simulink model "Masse_MultirotorSimHinf"  (R2018b)
settings: Solver=VariableStepAuto  StartTime=0.0  StopTime=Simulation.T_END  MaxStep=Simulation.TS_MAX  RelTol=1e-3  EnableMultiTasking=on
PreLoadFcn:
  | % InitializeParameters;
undefined symbols (not defined in the file): Aero, armed, ctrl_state, INIT_PARAM_VECTOR, Initial, K_i, K_p, Motor, mpc_att_sp, mpc_ctrl_state, mpc_manual, mpc_pos_sp_triplet, mpc_vehicle_land_detected, mpc_vehicle_status, Simulation, SOF1, SOF2, Uav, Upsilon, v_att_sp, v_control_mode
libraries: simulink_extras x9, simulink x6, dspstat3 x1, Px4Library x1
(part 1 of 11)
settings Model: PauseTimes=10.09  Creator=jban039  LastModifiedBy=jban039
settings DataIOCC: Decimation=10  ReturnWorkspaceOutputs=on  OutputOption=SpecifiedOutputTimes  OutputTimes=Simulation.T_OUT
settings OptimizationCC: LifeSpan=inf
settings DebuggingCC: ReadBeforeWriteMsg=DisableAll  WriteAfterWriteMsg=DisableAll  WriteAfterReadMsg=DisableAll  MultiTaskDSMMsg=none  UnconnectedLineMsg=none  AllowSymbolicDim=off  SFUnexpectedBacktrackingDiag=warning  SFNoUnconditionalDefaultTransitionDiag=warning  SFExecutionAtInitializationDiag=none
settings ModelReferenceCC: UpdateModelReferenceTargets=IfOutOfDate  ModelReferenceMinAlgLoopOccurrences=on  PropagateSignalLabelsOutOfModel=off
settings SFSimCC: SFSimEcho=off  SimUseLocalCustomCode=off
settings RTWCC: RTWUseLocalCustomCode=off
settings CodeAppCC: StateflowObjectComments=on
settings GRTTargetCC: TargetLangStandard=C89/C90 (ANSI)
settings ConfigComp: CovMetricSettings=dw  CovHtmlReporting=on  CovSaveCumulativeToWorkspaceVar=on  CovSaveSingleToWorkspaceVar=on  CovExternalEMLEnable=off

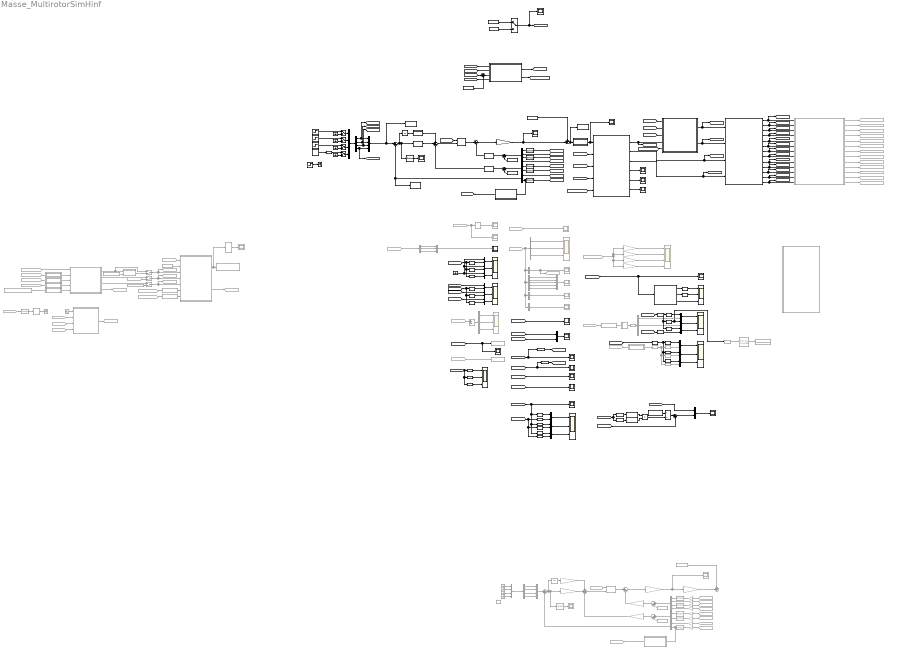
== system Masse_MultirotorSimHinf ==
  note: Important Notes
      |
      | NWU coordinate system used, therefore xBody faces forward, yBody faces to the left and zBody faces up
      | The UAV's state estimator, an extended kalman filter (referred to as LPE), is used for 3D position and velocity states.
      | PX4 rotor assignment: 1: front right, 2: back left, 3: front left, 4: back right
  note: Variables Description
      |
      | Variable
      | Vector notation
      | Frame
      | Description
      |
      | xi
      | [x y z]
      | World
      | Position
      |
      | eta
      | [phi theta psi]
      | World
      | Roll pitch yaw orientation
      |
      | nuBody
      | [p q r]
      | Body
      | Angular velocity
      |
      | q
      | [q1 q2 q3 q4]
      | World
      | Quaternion orientation
      |
      | Uav.BETA
      | [beta1 ... betaN]
      | Body
      | Angle to motor (CCW)
  note: Applied wind speed
  note: Inputs
  note: Scopes
  Acc : Scope  NumInputPorts=3
  Actuator controls : Scope  Commented=on
  Add : Sum  Commented=on  Inputs=+-
  Angular moments : Scope  NumInputPorts=3
  Angular rate integral : Scope  Commented=on  NumInputPorts=3
  Angular rates : Scope  NumInputPorts=3
  Applied body velocity : Scope
  Applied motor velocity : Scope  Commented=on  NumInputPorts=4
  Applied wind speed : Subsystem
  Attitude : Scope  NumInputPorts=3
  Attitude (quat) : Scope  Commented=on
  Bus Selector1 : BusSelector  Commented=on  OutputSignals=rates_sp
  Bus Selector10 : BusSelector  Commented=on  OutputSignals=mpc_local_pos_sp.acc_x,mpc_local_pos_sp.acc_y,mpc_local_pos_sp.acc_z
  Bus Selector2 : BusSelector  Commented=on  OutputSignals=controller_status.roll_rate_integ,controller_status.pitch_rate_integ,controller_status.yaw_rate_integ
  Bus Selector3 : BusSelector  Commented=on  OutputSignals=v_control_mode.flag_control_attitude_enabled,v_control_mode.flag_control_auto_enabled,v_control_mode.flag_control_manual_enabled,v_control_mode.flag_control_rates_enabled,v_control_mode.flag_control_velocity_enabled
  Bus Selector4 : BusSelector  Commented=on  OutputSignals=ctrl_state.q
  Bus Selector6 : BusSelector  Commented=on  OutputSignals=actuators.control
  Compute Sph : MATLAB Function  TreatAsAtomicUnit=on
  Constant : Constant  Value=Initial.U_M
  Constant1 : Constant  Value=abs(Uav.G(3))
  Constant2 : Constant  Value=Initial.Y2
  Constant3 : Constant  Value=Initial.Y1
  Constant4 : Constant  Commented=on  Value=Initial.U_M
  Constant5 : Constant  Commented=on  Value=Initial.Y2
  Constant6 : Constant  Commented=on  Value=Initial.Y1
  Default control stick positions : Constant  Commented=on  Value=[0; 0; 0.5; 0]
  Degrees to Radians : simulink_extras/Transformations/Degrees to Radians
  Degrees to Radians1 : simulink_extras/Transformations/Degrees to Radians  Commented=on
  Delay1 : Delay  Commented=on  DelayLength=1  SampleTime=1/10
  Demux : Demux  Commented=on  Outputs=3
  Demux1 : Demux
  Demux3 : Demux  Commented=on
  Demux6 : Demux  Commented=on  Outputs=3
  Desired accelerations : Scope
  Desired euler angles : Scope  Commented=on
  Desired quaternion : Scope  Commented=on
  Desired thrust : Scope  Commented=on
  Desired yaw rate : Scope
  Display : Display  Commented=on
  Divide : Product  Inputs=*/
  Divide1 : Product  Inputs=**
  Drag forces : Scope
  Drag model : ModelReference  ModelNameDialog=DragModelAIAAv3  SimulationMode=Normal  ModelReferenceVersion=1.368
  Drag moments : Scope
  Drag moments1 : Scope
  Fcn : Fcn  Expr=cos(u)
  Fcn1 : Fcn  Expr=cos(u)
  Fixed wind input : Constant  Value=[5.000000; 0.000000; 0]
  Flags : Scope  Commented=on
  From14 : From  Commented=on  GotoTag=attRateSp
  From16 : From  Commented=on  GotoTag=thrustDes
  From20 : From  Commented=on  GotoTag=posCtrlBus
  From21 : From  Commented=on  GotoTag=attCtrlBus
  From22 : From  Commented=on  GotoTag=qDes
  From34 : From  Commented=on  GotoTag=qDes
  From37 : From  Commented=on  GotoTag=VMotor_appBody
  From49 : From  Commented=on  GotoTag=R_star_bi
  From50 : From  Commented=on  GotoTag=xi
  From51 : From  Commented=on  GotoTag=eta
  From52 : From  Commented=on  GotoTag=xi
  From53 : From  Commented=on  GotoTag=xiDot
  From54 : From  Commented=on  GotoTag=nuBody
  From55 : From  Commented=on  GotoTag=xi
  From56 : From  Commented=on  GotoTag=xiDot
  From57 : From  Commented=on  GotoTag=eta
  From7 : From  Commented=on  GotoTag=eta
  From8 : From  Commented=on  GotoTag=xiMeasured
  Gain : Gain  Commented=on  Gain=[1;0;0;0]  Multiplication=Matrix(u*K)
  Gain1 : Gain  Commented=on  Gain=[0;1;0;0]  Multiplication=Matrix(u*K)
  Gain2 : Gain  Commented=on  Gain=[0;0;1;0]  Multiplication=Matrix(u*K)
  Gain3 : Gain  Commented=on  Gain=[0;0;0;1]  Multiplication=Matrix(u*K)
  Goto13 : Goto  Commented=on  GotoTag=VBodyMeasured
  Goto14 : Goto  Commented=on  GotoTag=VBodyDotMeasured
  Goto15 : Goto  Commented=on  GotoTag=qMeasured
  Goto16 : Goto  Commented=on  GotoTag=qDotMeasured
  Goto17 : Goto  Commented=on  GotoTag=qDDotMeasured
  Goto18 : Goto  Commented=on  GotoTag=nuBodyMeasured
  Goto19 : Goto  Commented=on  GotoTag=nuBodyDotMeasured
  Goto20 : Goto  Commented=on  GotoTag=xiMeasured
  Goto21 : Goto  Commented=on  GotoTag=xiDotMeasured
  Goto22 : Goto  Commented=on  GotoTag=xiDDotMeasured
  Goto23 : Goto  Commented=on  GotoTag=etaMeasured
  Goto24 : Goto  Commented=on  GotoTag=etaDotMeasured
  Goto25 : Goto  Commented=on  GotoTag=etaDDotMeasured
  Goto27 : Goto  Commented=on  GotoTag=R_star_bi
  Goto28 : Goto  Commented=on  GotoTag=attRateSp
  Ground{,5..8} (5 alike) : Ground  Commented=on
  Ground{1..4,9} (5 alike) : Ground
  Integrator1 : Integrator  Commented=on
  Integrator6 : Integrator
  K_i : Subsystem
      mask Display: fprintf('K_i')
  K_p : Subsystem
      mask Display: fprintf('K_p')
  Ki1 : Gain  Commented=on  Gain=K_i  Multiplication=Matrix(K*u)
  Kp1 : Gain  Commented=on  Gain=K_p  Multiplication=Matrix(K*u)
  Logging buffer : Subsystem
  MATLAB Function : MATLAB Function  TreatAsAtomicUnit=on
  MATLAB Function1 : MATLAB Function  Commented=on  TreatAsAtomicUnit=on
  Manual Switch{,1..3} (4 alike) : ManualSwitch
  Motor model : ModelReference  ModelNameDialog=MotorModelAIAAv3  SimulationMode=Normal  ModelReferenceVersion=1.394
  Motors - NED to NWU1 : Gain  Commented=on  Gain=[0 0 0 1; 0 0 1 0; 0 1 0 0; 1 0 0 0]  Multiplication=Matrix(K*u)
  Moving Average : dspstat3/Moving Average  Commented=on  Method=Sliding window  ForgettingFactorPort=off  SpecifyWindowLength=on  WindowLength=500  ForgettingFactor=0.9  SimulateUsing=Code generation
  Mux{,1,3,5..18,20..21} (19 alike) : Mux  Inputs=2
  Mux19 : Mux
  Mux2 : Mux  Commented=on  Inputs=5
  Mux22 : Mux
  Mux23 : Mux
  Mux24 : Mux  Commented=on  Inputs=2
  Mux25 : Mux  Commented=on
  Mux26 : Mux  Commented=on  Inputs=2
  Mux27 : Mux  Commented=on
  Mux28 : Mux  Commented=on
  Mux4 : Mux  Commented=on  Inputs=3
  NWU to NED Position1 : Subsystem  Commented=on  AncestorBlock=Px4Library/NWU to NED Position  mask(Coordinate transform){}
      mask help:
      | Convert a 3x1 vector or 4x1 quaternion from a North West Up to a North East Down coordinate system.
      |
      | The appropriate coordinate transform is automatically selected based on the input size.
  NWU to NED Quaternion3 : Subsystem  Commented=on  AncestorBlock=Px4Library/NWU to NED Quaternion  mask(Coordinate transform){}
      mask help:
      | Convert a 3x1 vector or 4x1 quaternion from a North West Up to a North East Down coordinate system.
      |
      | The appropriate coordinate transform is automatically selected based on the input size.
  NWU to NED{8..15} (8 alike) : Gain  Commented=on  Gain=[1 0 0; 0 -1 0; 0 0 -1]  Multiplication=Matrix(K*u)
  Omega : Scope
  Position tracking : Scope  NumInputPorts=3
  Product : Product  Multiplication=Matrix(*)
  Product1 : Product  Commented=on  Multiplication=Matrix(*)
  Quadcopter mixer : Px4Library/Quadcopter mixer  Commented=on  MC_SAMPLING_PERIOD=0.002
  Quadrotor Euler Model : Subsystem  Commented=on
  Quadrotor Quaternion Model : Subsystem
  Quaternion to Euler Angles : Subsystem  Commented=on  AncestorBlock=QuaternionLibrary/Quaternion to Euler Angles
      mask help: Convert an orientation quaternion to a vector of Euler angles
      mask Help:
      | Convert an orientation quaternion
      | [q1 q2 q3 q4]
      | where:
      | - q1 is the rotation in radians
      | - [q2 q3 q4] is the vector around which the rotation is performed)
      | to a vector of Euler angles
      | [roll, pitch, yaw]
      | Based on code from the PX4 firmware: https://github.com/PX4/Firmware
      mask Display: disp('Q2E')
  Quaternion to Euler Angles1 : Subsystem  Commented=on  AncestorBlock=QuaternionLibrary/Quaternion to Euler Angles
      mask help: Convert an orientation quaternion to a vector of Euler angles
      mask Help:
      | Convert an orientation quaternion
      | [q1 q2 q3 q4]
      | where:
      | - q1 is the rotation in radians
      | - [q2 q3 q4] is the vector around which the rotation is performed)
      | to a vector of Euler angles
      | [roll, pitch, yaw]
      | Based on code from the PX4 firmware: https://github.com/PX4/Firmware
      mask Display: disp('Q2E')
  Radians to Degrees{1..2,4..5,7} (5 alike) : simulink_extras/Transformations/Radians to Degrees
  Radians to Degrees3 : simulink_extras/Transformations/Radians to Degrees  Commented=on
  Radians to Degrees6 : simulink_extras/Transformations/Radians to Degrees  Commented=on
  Ramp : simulink/Sources/Ramp  slope=5  start=0  InitialOutput=0
  Rate setpoints : Scope  Commented=on
  SOF1 : Subsystem
      mask Display: fprintf('SOF1')
  SOF2 : Subsystem
      mask Display: fprintf('SOF2')
  SOF3 : Gain  Commented=on  Gain=SOF1  Multiplication=Matrix(K*u)
  SOF4 : Gain  Commented=on  Gain=SOF2  Multiplication=Matrix(K*u)
  Scope : Scope
  Scope1 : Scope  Commented=on
  Select Thrust : Selector  InputPortWidth=3  IndexOptions=Index vector (dialog)  Indices=[3]  OutputSizes=1
  Select pitch : Selector  InputPortWidth=3  IndexOptions=Index vector (dialog)  Indices=2  OutputSizes=1
  Select roll : Selector  InputPortWidth=3  IndexOptions=Index vector (dialog)  Indices=1  OutputSizes=1
  Select z : Selector  InputPortWidth=3  IndexOptions=Index vector (dialog)  Indices=[3]  OutputSizes=1
  Selector{,3,6,9,15,23..24} (7 alike) : Selector  InputPortWidth=3  IndexOptions=Index vector (dialog)  Indices=1  OutputSizes=1
  Selector{1,4,7,10,16,19,21} (7 alike) : Selector  InputPortWidth=3  IndexOptions=Index vector (dialog)  Indices=2  OutputSizes=1
  Selector{2,5,8,11,17,20,22,25,28..29} (10 alike) : Selector  InputPortWidth=3  IndexOptions=Index vector (dialog)  Indices=3  OutputSizes=1
  Selector12 : Selector  Commented=on  InputPortWidth=3  IndexOptions=Index vector (dialog)  Indices=2  OutputSizes=1
  Selector{13,31,34..35} (4 alike) : Selector  Commented=on  InputPortWidth=3  IndexOptions=Index vector (dialog)  Indices=3  OutputSizes=1
  Selector14 : Selector  Commented=on  InputPortWidth=3  IndexOptions=Index vector (dialog)  Indices=1  OutputSizes=1
  Selector18 : Selector  Commented=on  InputPortWidth=8  IndexOptions=Index vector (dialog)  Indices=[1 2 3]  OutputSizes=1
  Selector26 : Selector  InputPortWidth=3  IndexOptions=Index vector (dialog)  Indices=[2 1]  OutputSizes=1
  Selector27 : Selector  InputPortWidth=3  IndexOptions=Index vector (dialog)  Indices=[2 1]  OutputSizes=1
  Selector30 : Selector  InputPortWidth=4  IndexOptions=Index vector (dialog)  Indices=4  OutputSizes=1
  Selector32 : Selector  Commented=on  InputPortWidth=3  IndexOptions=Index vector (dialog)  Indices=[2 1]  OutputSizes=1
  Selector33 : Selector  Commented=on  InputPortWidth=3  IndexOptions=Index vector (dialog)  Indices=[2 1]  OutputSizes=1
  Selector36 : Selector  Commented=on  InputPortWidth=4  IndexOptions=Index vector (dialog)  Indices=4  OutputSizes=1
  Sensor Model : Subsystem  Commented=on
  Spherical body velocity : Scope  NumInputPorts=3
  Step : Step  Time=10  After=5  SampleTime=0
  Step1 : Step  Time=10  SampleTime=0
  Step2 : Step  Time=10  SampleTime=0
  Step3 : Step  Time=10  SampleTime=0
  Stick logging buffer : Subsystem  Commented=on
  Sum : Sum  Inputs=|++
  Sum1 : Sum  Inputs=++-
  Sum{10..13} (4 alike) : Sum  Commented=on  Inputs=|+-
  Sum2 : Sum  Inputs=++|
  Sum3 : Sum  Inputs=|++
  Sum{4..5,7..8} (4 alike) : Sum  Inputs=|+-
  Sum6 : Sum  Commented=on  Inputs=++-
  Sum9 : Sum  Commented=on  Inputs=++|
  TBody : Scope
  TBody1 : Scope
  TMotorIndividual : Scope
  Terminator : Terminator  Commented=on
  Terminator2 : Terminator
  Thust : Scope
  To Workspace : ToWorkspace  VariableName=r  SaveFormat=Timeseries  SampleTime=-1
  To Workspace eta : ToWorkspace  Commented=on  VariableName=eta  SaveFormat=Structure With Time  SampleTime=0.01
  To Workspace quat : ToWorkspace  Commented=on  VariableName=q  SaveFormat=Structure With Time  SampleTime=0.01
  To Workspace1 : ToWorkspace  VariableName=z  SaveFormat=Timeseries  SampleTime=-1
  To Workspace2 : ToWorkspace  VariableName=u_m  SaveFormat=Timeseries  SampleTime=-1
  Tracking error : Scope  Commented=on  NumInputPorts=3
  Upsilon : Gain  Gain=Upsilon  Multiplication=Matrix(K*u)
  Upsilon1 : Gain  Commented=on  Gain=Upsilon  Multiplication=Matrix(K*u)
  Varying wind input : FromWorkspace  VariableName=windInput  SampleTime=0
  Velocity tracking : Scope  NumInputPorts=3
  Wind Input : Scope
  Wind disturbance : Constant  Value=[0 0 0]
  Wind switch : ManualSwitch
  att_Goto_attCtrlBus : Goto  Commented=on  GotoTag=attCtrlBus
  att_Goto_thrustDes_ff : Goto  Commented=on  GotoTag=thrustDesFF
  att_NWUtoNED : Subsystem  Commented=on  AncestorBlock=Px4Library/NWU to NED Position  mask(Coordinate transform){}
      mask help:
      | Convert a 3x1 vector or 4x1 quaternion from a North West Up to a North East Down coordinate system.
      |
      | The appropriate coordinate transform is automatically selected based on the input size.
  att_PID_ff : simulink/Continuous/PID Controller  Commented=on  Controller=PID  Form=Parallel  TimeDomain=Continuous-time  SampleTime=-1  IntegratorMethod=Forward Euler  FilterMethod=Forward Euler  ControllerParametersSource=internal  P=-22.065410118279  I=-10.2297340963903  D=-11.7817329577601  UseFilter=on  N=104.897155810233  TunerSelectOption=Transfer Function Based (PID Tuner App)  InitialConditionSource=internal  InitialConditionForIntegrator=0  InitialConditionForFilter=0  DifferentiatorICPrevScaledInput=0  ExternalReset=none  TrackingMode=off  Kt=1  LimitOutput=off  UpperSaturationLimit=inf  LowerSaturationLimit=-inf  LinearizeAsGain=on  AntiWindupMode=none  Kb=1  POutMin=[]  POutMax=[]  IOutMin=[]  IOutMax=[]  DOutMin=[]  DOutMax=[]  NOutMin=[]  NOutMax=[]  SumOutMin=[]  SumOutMax=[]  SaturationOutMin=[]  SaturationOutMax=[]  PParamMin=[]  PParamMax=[]  IParamMin=[]  IParamMax=[]  DParamMin=[]  DParamMax=[]  NParamMin=[]  NParamMax=[]  KbParamMin=[]  KbParamMax=[]  KtParamMin=[]  KtParamMax=[]  KbOutMin=[]  KbOutMax=[]  KtOutMin=[]  KtOutMax=[]  IntegratorOutMin=[]  IntegratorOutMax=[]  FilterOutMin=[]  FilterOutMax=[]  SumI1OutMin=[]  SumI1OutMax=[]  SumI2OutMin=[]  SumI2OutMax=[]  SumI3OutMin=[]  SumI3OutMax=[]  SumI4OutMin=[]  SumI4OutMax=[]  SumDOutMin=[]  SumDOutMax=[]  DifferentiatorOutMin=[]  DifferentiatorOutMax=[]  FilterDiffOutCoefMin=[]  FilterDiffOutCoefMax=[]  ReciprocalOutMin=[]  ReciprocalOutMax=[]  SumDenOutMin=[]  SumDenOutMax=[]  SumNumOutMin=[]  SumNumOutMax=[]  DivideOutMin=[]  DivideOutMax=[]  IntegratorContinuousStateAttributes=''  IntegratorStateMustResolveToSignalObject=off  IntegratorRTWStateStorageClass=Auto  FilterContinuousStateAttributes=''  FilterStateMustResolveToSignalObject=off  FilterRTWStateStorageClass=Auto  ParallelPVariant=InternalParameters  IdealPVariant=Disabled  IVariant=InternalParameters  DVariant=InternalParameters  IntegratorVariant=Continuous  SatVariant=Disabled  AWVariant=Passthrough  PCopyVariant=Disabled  TRVariant=Disabled  FdbkBlocksVariant=Forward  IdealPFdbkVariant=Disabled  SatFdbkVariant=Disabled  DerivativeFilterVariant=ContFilter  NVariant=InternalParameters  NCopyVariant=Disabled  FilterICVariant=InternalICsFilter  IntegratorICVariant=InternalICs  ExternalResetVariant=Disabled  TRSumVariant=Passthrough  SumFdbkVariant=Disabled  SumVariant=Sum_PID
  att_controller_ff : MATLAB Function  Commented=on  TreatAsAtomicUnit=on
  att_flags : Constant  Commented=on  Value=[1, 0, 1, 1, 1]
  att_from_VappBody_ff : From  Commented=on  GotoTag=V_appBody
  att_from_armed : From  Commented=on  GotoTag=armed
  att_from_nuBody : From  Tag=nuBody  Commented=on  GotoTag=nuBody
  att_from_omega_ff : From  Commented=on  GotoTag=omega
  att_from_q : From  Tag=q  Commented=on  GotoTag=q
  att_from_q_ff : From  Commented=on  GotoTag=q
  att_from_thrustDesFF_ff : From  Commented=on  GotoTag=thrustDesFF
  att_mixerInput : Subsystem  Commented=on
  att_qDesInput : FromWorkspace  Commented=on  VariableName=AttInput.qDes  SampleTime=0  Interpolate=off  OutputAfterFinalValue=Holding final value
  att_qDesSwitch : ManualSwitch  Commented=on  CurrentSetting=0
  att_q_NWUtoNED : Subsystem  Commented=on  AncestorBlock=Px4Library/NWU to NED Quaternion  mask(Coordinate transform){}
      mask help:
      | Convert a 3x1 vector or 4x1 quaternion from a North West Up to a North East Down coordinate system.
      |
      | The appropriate coordinate transform is automatically selected based on the input size.
  att_selector_ff : Selector  Commented=on  InputPortWidth=3  IndexOptions=Index vector (dialog)  Indices=3  OutputSizes=1
  att_thrustDesSwitch : ManualSwitch  Commented=on  CurrentSetting=0
  att_xi_ff : From  Commented=on  GotoTag=xi
  att_yawRateDesInput : FromWorkspace  Commented=on  VariableName=AttInput.yawRateDes  SampleTime=0  Interpolate=off  OutputAfterFinalValue=Holding final value
  att_yawRateDesSwitch : ManualSwitch  Commented=on  CurrentSetting=0
  mc_att_control : Subsystem  Commented=on  AncestorBlock=Px4Library/mc_att_control  mask(PX4 Attitude Controller: mc_att_control){MC_SAMPLING_PERIOD=0.004, MC_ROLL_TC=0.2, MC_PITCH_TC=0.2, MC_ROLL_P=6.5, MC_ROLLRATE_P=0.15, MC_ROLLRATE_I=0.05, MC_ROLLRATE_D=0.003, MC_ROLLRATE_FF=0, MC_PITCH_P=6.5, MC_PITCHRATE_P=0.15, MC_PITCHRATE_I=0.05, MC_PITCHRATE_D=0.003, MC_PITCHRATE_FF=0, MC_YAW_P=2.8, MC_YAWRATE_P=0.2, MC_YAWRATE_I=0.1, MC_YAWRATE_D=0, MC_YAWRATE_FF=0, MC_YAW_FF=0.5, MC_ROLLRATE_MAX=220, MC_PITCHRATE_MAX=220, MC_YAWRATE_MAX=200, MC_YAWRAUTO_MAX=45, MC_ACRO_R_MAX=360, MC_ACRO_P_MAX=360, MC_ACRO_Y_MAX=360, MC_RATT_TH=1, MC_TPA_BREAK=1, MC_TPA_SLOPE=1, VT_OPT_RECOV_EN=0, VT_WV_YAWR_SCL=0.15, MC_RR_INT_LIM=0.30, MC_PR_INT_LIM=0.30, MC_TPA_BREAK_P=1.0, MC_TPA_BREAK_I=1.0, MC_TPA_BREAK_D=1.0, MC_TPA_RATE_P=0.0, MC_TPA_RATE_I=0.0, MC_TPA_RATE_D=0.0, VT_TYPE=0, MC_BAT_SCALE_EN=0, MC_YR_INT_LIM=0.30}
      mask prompts: VT_TYPE "VT_TYPE (0 = Tailsitter, 1 = Tiltrotor, 2 = Standard)"
      mask help: Stabilization controller from the PX4 flight stack.
  mc_pos_control : Subsystem  Commented=on  AncestorBlock=Px4Library/mc_pos_control  mask{THROTTLE_HOVER=Uav.THROTTLE_HOVER, MPC_SAMPLING_PERIOD=0.02, MPC_THR_MIN=0.12, MPC_THR_HOVER=0.5, MPC_ALTCTL_DZ=0.1, MPC_ALTCTL_DY=0, MPC_THR_MAX=0.9, MPC_MANTHR_MIN=0.08, MPC_MANTHR_MAX=0.9, MPC_Z_P=1, MPC_Z_VEL_P=0.2, MPC_Z_VEL_I=0.02, MPC_Z_VEL_D=0, MPC_Z_VEL_MAX_UP=3, MPC_Z_VEL_MAX=1, MPC_Z_VEL_MAX_DN=1, MPC_Z_FF=0.5, MPC_XY_P=0.95, MPC_XY_VEL_P=0.09, MPC_XY_VEL_I=0.02, MPC_XY_VEL_D=0.01, MPC_XY_CRUISE=5, MPC_XY_VEL_MAX=8, MPC_XY_FF=0.5, MPC_TILTMAX_AIR=45, MPC_TILTMAX_LND=12, MPC_LAND_SPEED=0.5, MPC_TKO_SPEED=1.5, MPC_MAN_R_MAX=35, MPC_MAN_P_MAX=35, MPC_MAN_Y_MAX=200, MPC_HOLD_XY_DZ=0.1, MPC_HOLD_MAX_XY=0.8, MPC_HOLD_MAX_Z=0.6, MPC_VELD_LP=5, MPC_ACC_HOR_MAX=5, MPC_ALT_MODE=1, MC_YAWRATE_MAX=200, MC_YAW_P=2.8, VT_OPT_RECOV_EN=0}
      mask init:
      | throttle_hover = THROTTLE_HOVER; % evalin('base', THROTTLE_HOVER);
      | MPC_INIT_SELF = struct( 'mpc_param_find', struct( ...
      | 'MC_YAWRATE_MAX', MC_YAWRATE_MAX, ...
      | 'MC_YAW_P', MC_YAW_P, ...
      | 'MPC_ACC_HOR_MAX', MPC_ACC_HOR_MAX, ...
      | 'MPC_ALTCTL_DY', MPC_ALTCTL_DY, ...
      | 'MPC_ALTCTL_DZ', MPC_ALTCTL_DZ, ...
      | 'MPC_ALT_MODE', MPC_ALT_MODE, ...
      | 'MPC_HOLD_MAX_XY', MPC_HOLD_MAX_XY, ...
      | 'MPC_HOLD_MAX_Z', MPC_HOLD_MAX_Z, ...
      | 'MPC_HOLD_XY_DZ', MPC_HOLD_XY_DZ, ...
      | 'MPC_LAND_SPEED', MPC_LAND_SPEED, ...
      | 'MPC_MAN_P_MAX', MPC_MAN_P_MAX, ...
      | 'MPC_MAN_R_MAX', MPC_MAN_R_MAX, ...
      | 'MPC_MAN_Y_MAX', MPC_MAN_Y_MAX, ...
      | 'MPC_THR_HOVER', MPC_THR_HOVER, ...
      | 'MPC_THR_MAX', MPC_THR_MAX, ...
      | 'MPC_THR_MIN', MPC_THR_MIN, ...
      | 'MPC_TILTMAX_AIR', MPC_TILTMAX_AIR, ...
      | 'MPC_TILTMAX_LND', MPC_TILTMAX_LND, ...
      | 'MPC_TKO_SPEED', MPC_TKO_SPEED, ...
      | 'MPC_XY_CRUISE', MPC_XY_CRUISE, ...
      | 'MPC_XY_FF', MPC_XY_FF, ...
      | 'MPC_XY_P', MPC_XY_P, ...
      | 'MPC_XY_VEL_D', MPC_XY_VEL_D, ...
      | 'MPC_XY_VEL_I', MPC_XY_VEL_I, ...
      | 'MPC_XY_VEL_MAX', MPC_XY_VEL_MAX, ...
      | 'MPC_XY_VEL_P', MPC_XY_VEL_P, ...
      | 'MPC_Z_FF', MPC_Z_FF, ...
      | 'MPC_Z_P', MPC_Z_P, ...
      | 'MPC_Z_VEL_D', MPC_Z_VEL_D, ...
      | 'MPC_Z_VEL_I', MPC_Z_VEL_I, ...
      | 'MPC_Z_VEL_MAX', MPC_Z_VEL_MAX, ...
      | 'MPC_Z_VEL_MAX_DN', MPC_Z_VEL_MAX_DN, ...
      | 'MPC_Z_VEL_MAX_UP', MPC_Z_VEL_MAX_UP, ...
      | 'MPC_Z_VEL_P', MPC_Z_VEL_P, ...
      | 'VT_OPT_RECOV_EN', VT_OPT_RECOV_EN, ...
      | 'MPC_VELD_LP', MPC_VELD_LP ...
      | ), ...
      | 'mpc_thrust_int', [0; 0; -throttle_hover], ...
      | 'mpc_att_sp', struct('thrust', throttle_hover, ...
      | 'q_d', [1; 0; 0; 0;]) ...
      | );
  pos_Goto_posCtrlBus : Goto  Commented=on  GotoTag=posCtrlBus
  pos_Goto_qDes : Goto  Commented=on  GotoTag=qDes
  pos_Goto_thrustDes : Goto  Commented=on  GotoTag=thrustDes
  pos_Goto_yawRateDes : Goto  Commented=on  GotoTag=yawRateDes
  pos_NWUtoNED1 : Subsystem  Commented=on  AncestorBlock=Px4Library/NWU to NED Position  mask(Coordinate transform){}
      mask help:
      | Convert a 3x1 vector or 4x1 quaternion from a North West Up to a North East Down coordinate system.
      |
      | The appropriate coordinate transform is automatically selected based on the input size.
  pos_NWUtoNED2 : Subsystem  Commented=on  AncestorBlock=Px4Library/NWU to NED Position  mask(Coordinate transform){}
      mask help:
      | Convert a 3x1 vector or 4x1 quaternion from a North West Up to a North East Down coordinate system.
      |
      | The appropriate coordinate transform is automatically selected based on the input size.
  pos_from_armed : From  Commented=on  GotoTag=armed
  pos_from_q : From  Tag=q  Commented=on  GotoTag=q
  pos_from_xi : From  Tag=xi  Commented=on  GotoTag=xi
  pos_from_xiDot : From  Tag=xiDot  Commented=on  GotoTag=xiDot
  pos_q_NWUtoNED : Subsystem  Commented=on  AncestorBlock=Px4Library/NWU to NED Quaternion  mask(Coordinate transform){}
      mask help:
      | Convert a 3x1 vector or 4x1 quaternion from a North West Up to a North East Down coordinate system.
      |
      | The appropriate coordinate transform is automatically selected based on the input size.
  pwm : Scope
  pwm1 : Scope  Commented=on
  pwm2 : Scope
  pwm3 : Scope  Commented=on
  q : Scope
  realPwm : Scope
  tauMotorIndividual1 : Scope
  wires:
  Motor model/1 -> [omega], Drag model/4  "omega"
  Motor model/2 -> Quadrotor Quaternion Model/3(TBody), [TBody]  "TBody"
  Drag model/2 -> Quadrotor Quaternion Model/2(M_DBody), [M_D]  "M_D"
  Quadrotor Quaternion Model/1(VBody) -> Sensor Model/1(VBody), [VBody]  "VBody"
  Quadrotor Quaternion Model/2(VBodyDot) -> Sensor Model/2(VBodyDot), [VBodyDot]  "VBodyDot"
  Quadrotor Quaternion Model/3(nuBody) -> Sensor Model/3(nuBody), [nuBody]  "nuBody"
  Quadrotor Quaternion Model/4(nuBodyDot) -> Sensor Model/4(nuBodyDot), [nuBodyDot]  "nuBodyDot"
  Quadrotor Quaternion Model/5(xi) -> Sensor Model/5(xi), [xi]  "xi"
  Quadrotor Quaternion Model/6(xiDot) -> Sensor Model/6(xiDot), [xiDot]  "xiDot"
  Quadrotor Quaternion Model/7(xiDDot) -> Sensor Model/7(xiDDot), [xiDDot]  "xiDDot"
  Quadrotor Quaternion Model/8(eta) -> Sensor Model/8(eta), [eta]  "eta"
  Quadrotor Quaternion Model/9(etaDot) -> Sensor Model/9(etaDot), [etaDot]  "etaDot"
  Quadrotor Quaternion Model/10(etaDDot) -> Sensor Model/10(etaDDot), [etaDDot]  "etaDDot"
  [V_appBody] -> Drag model/2
  [nuBody] -> Motor model/2
  Quadrotor Quaternion Model/11(q) -> Sensor Model/11(q), [q]  "q"
  Quadrotor Quaternion Model/12(qDot) -> Sensor Model/12(qDot), [qDot]  "qDot"
  Quadrotor Quaternion Model/13(qDDot) -> Sensor Model/13(qDDot), [qDDot]  "qDDot"
  Drag model/1 -> Quadrotor Quaternion Model/1(F_DBody), [F_D]  "F_D"
  Sensor Model/1(VBodyMeasured) -> Goto13/1
  Sensor Model/2(VBodyDotMeasured) -> Goto14/1
  Sensor Model/3(nuBodyMeasured) -> Goto18/1
  Sensor Model/4(nuBodyDotMeasured) -> Goto19/1
  Sensor Model/5(xiMeasured) -> Goto20/1  "xiMeasured"
  Sensor Model/6(xiDotMeasured) -> Goto21/1  "xiDotMeasured"
  Sensor Model/7(xiDDotMeasured) -> Goto22/1
  Sensor Model/8(etaMeasured) -> Goto23/1
  Sensor Model/9(etaDotMeasured) -> Goto24/1
  Sensor Model/10(etaDDotMeasured) -> Goto25/1
  Sensor Model/11(qMeasured) -> Goto15/1  "qMeasured"
  Sensor Model/12(qDotMeasured) -> Goto16/1
  Sensor Model/13(qDDotMeasured) -> Goto17/1
  Logging buffer/1(pwmOut) -> pwm/1, Motor model/1  "pwm"
  att_from_nuBody/1 -> att_NWUtoNED/1(posNWU)
  Bus Selector2/1 -> Angular rate integral/1  "<roll_rate_integ>"
  Bus Selector2/2 -> Angular rate integral/2  "<pitch_rate_integ>"
  Bus Selector2/3 -> Angular rate integral/3  "<yaw_rate_integ>"
  From21/1 -> Bus Selector2/1, Bus Selector1/1, Bus Selector6/1, Bus Selector4/1, Bus Selector3/1
  Bus Selector1/1 -> Goto28/1, Rate setpoints/1  "<rates_sp>"
  Bus Selector3/1 -> Mux2/1  "<flag_control_attitude_enabled>"
  Bus Selector3/2 -> Mux2/2  "<flag_control_auto_enabled>"
  Bus Selector3/3 -> Mux2/3  "<flag_control_manual_enabled>"
  Bus Selector3/4 -> Mux2/4  "<flag_control_rates_enabled>"
  Bus Selector3/5 -> Mux2/5  "<flag_control_velocity_enabled>"
  Mux2/1 -> Flags/1
  Bus Selector4/1 -> Attitude (quat)/1  "<q>"
  Bus Selector6/1 -> Actuator controls/1  "<control>"
  From20/1 -> Bus Selector10/1
  pos_from_q/1 -> pos_q_NWUtoNED/1(qNWU)
  Stick logging buffer/1(stickOut) -> mc_pos_control/5(stick)  "stickPos"
  att_from_q/1 -> att_q_NWUtoNED/1(qNWU)
  att_q_NWUtoNED/1(qNED) -> mc_att_control/6(q)
  att_NWUtoNED/1(posNED) -> mc_att_control/7(nuBody)
  pos_q_NWUtoNED/1(qNED) -> mc_pos_control/2(qNED)
  mc_pos_control/3(yawRateDes) -> att_yawRateDesSwitch/1
  att_controller_ff/1(thrustDes) -> att_Goto_thrustDes_ff/1
  pos_NWUtoNED1/1(posNED) -> mc_pos_control/4(velNED)
  pos_NWUtoNED2/1(posNED) -> mc_pos_control/3(posNED)
  pos_from_xi/1 -> pos_NWUtoNED2/1(posNWU)
  Bus Selector10/1 -> Mux4/1  "<acc_x>"
  Bus Selector10/2 -> Mux4/2  "<acc_y>"
  Bus Selector10/3 -> Mux4/3  "<acc_z>"
  Mux4/1 -> Desired accelerations/1
  Selector6/1 -> Mux6/1  "act_r"
  Selector7/1 -> Delay1/1, Mux5/1  "act_p"
  Mux7/1 -> Velocity tracking/3
  Mux8/1 -> Velocity tracking/2
  Mux9/1 -> Velocity tracking/1
  Ground9/1 -> Mux9/1, Mux8/1, Mux7/1  "vel_sp_x"
  Selector/1 -> Mux9/2  "vel_x"
  Selector1/1 -> Mux8/2  "vel_y"
  Selector2/1 -> Mux7/2  "vel_z"
  Mux10/1 -> Position tracking/3
  Mux11/1 -> Position tracking/2
  Mux12/1 -> Position tracking/1
  [xDes] -> Mux12/1  "sp_x"
  Selector3/1 -> Mux12/2  "meas_x"
  [yDes] -> Mux11/1  "sp_y"
  Selector4/1 -> Mux11/2  "meas_y"
  [zDes] -> Mux10/1  "sp_z"
  Selector5/1 -> Mux10/2  "meas_z"
  Quaternion to Euler Angles/1(euler) -> Radians to Degrees3/1
  Demux6/1 -> Mux6/2  "sp_r"
  Demux6/2 -> Mux5/2  "sp_p"
  Radians to Degrees7/1 -> Mux1/2  "sp_y"
  Selector8/1 -> Mux1/1  "act_y"
  NWU to NED Quaternion3/1(qNED) -> Quaternion to Euler Angles/1(quaternion)
  mc_att_control/1(actuatorsControl) -> Selector18/1, Quadcopter mixer/1
  Upsilon/1 -> Sum2/2, pwm2/1  "u_m"
  Add/1 -> Demux/1
  Demux/1 -> Tracking error/1  "posTrackingX"
  Demux/2 -> Tracking error/2  "posTrackingY"
  Demux/3 -> Tracking error/3  "posTrackingZ"
  [nuBody] -> Drag model/3
  Mux6/1 -> Attitude/1  "roll"
  Mux5/1 -> Attitude/2  "pitch"
  [eta] -> Motor model/3
  [q] -> q/1, To Workspace quat/1
  From7/1 -> To Workspace eta/1
  [xiDot] -> Selector2/1, Selector1/1, Selector/1
  [xi] -> Selector5/1, Selector4/1, Selector3/1
  From8/1 -> Add/1
  Wind switch/1 -> [windInput], Wind Input/1  "windInput"
  [V_appBody] -> Motor model/4
  att_flags/1 -> mc_att_control/2(flags)  "mcFlags"
  mc_pos_control/4(bus) -> pos_Goto_posCtrlBus/1  "posCtrlBus"
  mc_att_control/2(bus) -> att_Goto_attCtrlBus/1  "attCtrlBus"
  From22/1 -> NWU to NED Quaternion3/1(qNWU)
  att_from_armed/1 -> mc_att_control/1(armed)
  pos_from_armed/1 -> mc_pos_control/1(armed)
  Fixed wind input/1 -> Wind switch/2
  Varying wind input/1 -> Wind switch/1
  [omega] -> Omega/1
  Radians to Degrees3/1 -> Demux6/1
  Radians to Degrees4/1 -> Selector8/1, Selector7/1, Selector6/1
  [eta] -> Radians to Degrees4/1
  Motor model/4 -> TMotorIndividual/1
  [thrustDes] -> Mux3/1
  [thrustBody] -> Mux3/2
  Mux3/1 -> Thust/1
  Motor model/5 -> tauMotorIndividual1/1
  [xi] -> Drag model/1
  pos_from_xiDot/1 -> pos_NWUtoNED1/1(posNWU)
  [TBody] -> Select Thrust/1, TBody/1  "TBody"
  Select Thrust/1 -> [thrustBody]
  [F_D] -> Drag forces/1, Select z/1
  [V_appBody] -> Compute Sph/1(V_appBody), Applied body velocity/1
  Compute Sph/1(azimuth) -> Radians to Degrees1/1
  Compute Sph/2(elevation) -> Radians to Degrees2/1
  Compute Sph/3(radius) -> Spherical body velocity/3
  Radians to Degrees1/1 -> Spherical body velocity/1
  Radians to Degrees2/1 -> Spherical body velocity/2
  [M_D] -> Drag moments/1
  [VMotor_appBody] -> Motor model/5
  From37/1 -> Gain3/1, Gain2/1, Gain/1, Gain1/1
  Gain/1 -> Applied motor velocity/1
  Gain1/1 -> Applied motor velocity/2
  Gain2/1 -> Applied motor velocity/3
  Gain3/1 -> Applied motor velocity/4
  [VMotor_appBody] -> Drag model/5
  att_qDesSwitch/1 -> pos_Goto_qDes/1, mc_att_control/3(qDes)  "qDes"
  att_thrustDesSwitch/1 -> pos_Goto_thrustDes/1, mc_att_control/4(thrustDes)  "thrustDes"
  att_yawRateDesSwitch/1 -> pos_Goto_yawRateDes/1, mc_att_control/5(yawRateDes)  "yawRateDes"
  att_yawRateDesInput/1 -> att_yawRateDesSwitch/2
  att_from_thrustDesFF_ff/1 -> att_thrustDesSwitch/2
  [yawRateDes] -> Desired yaw rate/1
  Mux1/1 -> Attitude/3  "yaw"
  Motor model/3 -> Quadrotor Quaternion Model/4(tauBody), [tauBody]  "tauBody"
  [VBody] -> Applied wind speed/1(VBody)
  [q] -> Applied wind speed/2(q)
  [windInput] -> Sum/1
  Applied wind speed/1(V_appBody) -> [V_appBody]
  Applied wind speed/2(VMotor_appBody) -> [VMotor_appBody]
  [nuBody] -> Applied wind speed/4(nuBody)
  Selector9/1 -> Mux15/1  "act_r"
  Selector10/1 -> Mux14/1  "act_p"
  Selector11/1 -> Mux13/1  "act_y"
  Mux15/1 -> Angular rates/1
  Mux14/1 -> Angular rates/2
  Radians to Degrees5/1 -> Selector9/1, Selector11/1, Selector10/1
  [nuBody] -> Radians to Degrees5/1
  Mux13/1 -> Angular rates/3
  Radians to Degrees6/1 -> Selector14/1, Selector13/1, Selector12/1
  Selector14/1 -> Mux15/2  "sp_r"
  Selector12/1 -> Mux14/2  "sp_p"
  Selector13/1 -> Mux13/2  "sp_y"
  From14/1 -> NWU to NED Position1/1(posNWU)
  NWU to NED Position1/1(posNED) -> Radians to Degrees6/1
  Selector15/1 -> Acc/1  "acc_x"
  Selector16/1 -> Acc/2  "acc_y"
  Selector17/1 -> Acc/3  "acc_z"
  [xiDDot] -> Selector15/1, Selector16/1, Selector17/1
  From16/1 -> Desired thrust/1
  Selector18/1 -> pwm1/1
  [M_D] -> Selector20/1, Selector19/1, Selector24/1, Drag moments1/1
  Mux18/1 -> Angular moments/1
  Mux17/1 -> Angular moments/2
  Mux16/1 -> Angular moments/3
  Selector24/1 -> Mux18/1  "dragX"
  Selector23/1 -> Mux18/2  "motorX"
  Selector19/1 -> Mux17/1  "dragY"
  Selector21/1 -> Mux17/2  "motorY"
  Selector20/1 -> Mux16/1  "dragZ"
  Selector22/1 -> Mux16/2  "MotorZ"
  [tauBody] -> Selector22/1, Selector21/1, Selector23/1
  Default control stick positions/1 -> Stick logging buffer/1(stickIn)
  From34/1 -> Desired quaternion/1, Quaternion to Euler Angles1/1(quaternion)
  Quaternion to Euler Angles1/1(euler) -> Desired euler angles/1  "etaDes"
  att_from_VappBody_ff/1 -> att_controller_ff/2(V_appBody)
  att_selector_ff/1 -> att_PID_ff/1
  att_xi_ff/1 -> att_selector_ff/1
  att_from_q_ff/1 -> att_controller_ff/3(q)
  att_from_omega_ff/1 -> att_controller_ff/4(omega)
  Divide/1 -> Sum3/1
  Sum3/1 -> Mux21/2  "thrustRequired"
  Mux21/1 -> TBody1/1
  Constant1/1 -> Divide/1
  Select z/1 -> [F_Dz]
  [thrustBody] -> Mux21/1
  [eta] -> Select pitch/1, Select roll/1
  Select roll/1 -> Fcn/1
  Select pitch/1 -> Fcn1/1
  Fcn/1 -> Divide1/1
  Fcn1/1 -> Divide1/2
  Divide1/1 -> Divide/2
  [F_Dz] -> Sum3/2
  mc_pos_control/1(qDes) -> att_qDesSwitch/1, att_mixerInput/1(qPosCtrl)
  mc_pos_control/2(thrustDes) -> att_thrustDesSwitch/1
  att_mixerInput/1(qDes) -> att_qDesSwitch/2
  att_qDesInput/1 -> att_mixerInput/2(qInput)
  Delay1/1 -> Moving Average/1
  Moving Average/1 -> Display/1
  att_PID_ff/1 -> Terminator/1
  Ground/1 -> att_controller_ff/1(Textra)
  Demux1/4 -> [psiDes], Mux19/4  "psi_d"
  Demux1/1 -> [xDes], Mux19/1  "x_d"
  Demux1/3 -> [zDes], Mux19/3  "z_d"
  Demux1/2 -> [yDes], Mux19/2  "y_d"
  Mux23/1 -> Demux1/1  "r"
  K_i/1(u) -> Sum1/1  "k_i*int(e)"
  Sum1/1 -> Product/2  "u_i_v"
  Mux19/1 -> Sum8/1, To Workspace/1  "r"
  Sum7/1 -> Upsilon/1  "u_v"
  [R_star_bi] -> Product/1
  Product/1 -> Sum7/1  "u_b_v"
  Mux/1 -> To Workspace1/1, Sum8/2  "z"
  Sum8/1 -> Integrator6/1, K_p/1(e), Selector30/1  "e"
  SOF1/1(u1) -> Sum1/3
  Integrator6/1 -> K_i/1(int(e))  "int(e)"
  K_p/1(u) -> Sum1/2  "k_p*e"
  [xi] -> Mux/1  "xi"
  Selector25/1 -> MATLAB Function/1(psi), Mux/2  "psi"
  Selector27/1 -> Mux20/2
  Selector26/1 -> Mux20/1
  Sum5/1 -> SOF1/1(y1)
  Selector28/1 -> Mux22/1
  Selector29/1 -> Mux22/3
  MATLAB Function/1(R_star_bi) -> [R_star_bi]
  Sum/1 -> Applied wind speed/3(U)
  Wind disturbance/1 -> Sum/2  "w"
  Sum2/1 -> To Workspace2/1, Logging buffer/1(pwmIn)
  Constant/1 -> Sum2/1
  Mux22/1 -> Sum4/1
  Mux20/1 -> Sum5/1
  Constant2/1 -> Sum4/2
  Constant3/1 -> Sum5/2
  Ramp/1 -> Degrees to Radians/1
  Selector30/1 -> Scope/1
  [eta] -> Selector25/1
  [xi] -> Selector27/1
  [xiDot] -> Selector26/1
  [eta] -> Mux22/4
  [xi] -> Selector29/1
  [nuBody] -> Mux22/2
  [xiDot] -> Selector28/1
  SOF4/1 -> Sum12/2
  Ground6/1 -> Mux28/3
  Constant5/1 -> Sum10/2
  Mux26/1 -> Sum11/1
  Constant4/1 -> Sum9/1
  Constant6/1 -> Sum11/2
  Ground5/1 -> Mux28/1
  Selector34/1 -> Mux27/1
  Sum10/1 -> SOF4/1
  From54/1 -> NWU to NED14/1
  Selector35/1 -> Mux27/3
  Selector33/1 -> Mux26/2
  Sum6/1 -> Product1/2  "u_i_v"
  Demux3/4 -> Mux25/4  "psi_d"
  Sum13/1 -> Integrator1/1, Selector36/1, Kp1/1  "e"
  From50/1 -> NWU to NED9/1  "xi"
  Ground7/1 -> Mux28/2
  MATLAB Function1/1(R_star_bi) -> Goto27/1
  Mux24/1 -> Sum13/2  "z"
  From53/1 -> NWU to NED11/1
  Demux3/2 -> Mux25/2  "y_d"
  Selector32/1 -> Mux26/1
  Integrator1/1 -> Ki1/1
  Demux3/3 -> Mux25/3  "z_d"
  From52/1 -> NWU to NED10/1
  Product1/1 -> Sum12/1  "u_b_v"
  Selector31/1 -> MATLAB Function1/1(psi), Mux24/2  "psi"
  ? -> Degrees to Radians1/1
  Ground8/1 -> Mux28/4
  Selector36/1 -> Scope1/1
  NWU to NED11/1 -> Selector32/1
  Demux3/1 -> Mux25/1  "x_d"
  NWU to NED10/1 -> Selector33/1
  From56/1 -> NWU to NED15/1
  Upsilon1/1 -> Motors - NED to NWU1/1, pwm3/1  "u_m"
  From57/1 -> NWU to NED12/1
  From51/1 -> NWU to NED8/1
  Motors - NED to NWU1/1 -> Sum9/2
  Ki1/1 -> Sum6/1  "k_i*xi"
  Sum11/1 -> SOF3/1
  From55/1 -> NWU to NED13/1
  Sum12/1 -> Upsilon1/1  "u_v"
  Mux27/1 -> Sum10/1
  NWU to NED15/1 -> Selector34/1
  NWU to NED12/1 -> Mux27/4
  NWU to NED8/1 -> Selector31/1
  SOF3/1 -> Sum6/3
  Kp1/1 -> Sum6/2  "k_p*e"
  From49/1 -> Product1/1
  NWU to NED13/1 -> Selector35/1
  Mux25/1 -> Sum13/1  "r"
  NWU to NED14/1 -> Mux27/2
  NWU to NED9/1 -> Mux24/1
  Mux28/1 -> Demux3/1  "r"
  Step1/1 -> Manual Switch/1
  Sum4/1 -> SOF2/1(y2)
  SOF2/1(u2) -> Sum7/2
  Step/1 -> Terminator2/1
  [psiDes] -> Radians to Degrees7/1
  Manual Switch/1 -> Mux23/1
  Manual Switch1/1 -> Mux23/2
  Manual Switch2/1 -> Mux23/3
  Manual Switch3/1 -> Mux23/4
  Ground1/1 -> Manual Switch3/2
  Degrees to Radians/1 -> Manual Switch3/1
  Ground2/1 -> Manual Switch2/2
  Ground3/1 -> Manual Switch1/2
  Ground4/1 -> Manual Switch/2
  Step2/1 -> Manual Switch1/1
  Step3/1 -> Manual Switch2/1
  Motor model/6 -> realPwm/1

== system Masse_MultirotorSimHinf/Applied wind speed ==
  VBody : Inport  Unit=m/s
  q : Inport  Port=2
  U : Inport  Port=3  Unit=m/s
  nuBody : Inport  Port=4  Unit=rad/s
  Compute V_app2 : MATLAB Function  TreatAsAtomicUnit=on
  Gain : Gain  Gain=ones(1,Uav.N_ROTORS)  Multiplication=Matrix(u*K)
  Gain1 : Gain  Gain=ones(1,Uav.N_ROTORS)  Multiplication=Matrix(u*K)
  Quaternion to Rotation Matrix1 : Subsystem  AncestorBlock=QuaternionLibrary/Quaternion to Rotation Matrix
      mask help: Convert an orientation quaternion to an orthogonal transformation matrix
      mask Help:
      | Convert an orientation quaternion
      | [q1 q2 q3 q4]
      | where:
      | - q1 is the rotation in radians
      | - [q2 q3 q4] is the vector around which the rotation is performed)
      | to an orthogonal transformation matrix
      | Based on code from the PX4 firmware: https://github.com/PX4/Firmware
      mask Display: disp('Q2R')
  Relative velocities : Scope
  Relative velocity : MATLAB Function  TreatAsAtomicUnit=on
  Rotational velocities : Scope
  Sum : Sum  Inputs=++|
  Sum1 : Sum  Inputs=++|
  V_appBody : Outport  Unit=m/s
  VMotor_appBody : Outport  Port=2  Unit=m/s  PortDimensions=[3,Uav.N_ROTORS]
  wires:
  Gain1/1 -> Relative velocity/1(nuBody)
  Sum1/1 -> V_appBody/1, Gain/1
  Compute V_app2/1(UBody) -> Sum1/2
  Relative velocity/1(VMotorRelBody) -> Sum/2, Relative velocities/1
  q/1 -> Quaternion to Rotation Matrix1/1(quaternion)
  VBody/1 -> Sum1/1
  Gain/1 -> Sum/1
  nuBody/1 -> Rotational velocities/1, Gain1/1
  Quaternion to Rotation Matrix1/1(rotationMatrix) -> Compute V_app2/1(Q)
  Sum/1 -> VMotor_appBody/1  "VMotorBody"
  U/1 -> Compute V_app2/2(U)

== system Masse_MultirotorSimHinf/K_i ==
  int(e) : Inport
  Demux : Demux
  Demux1 : Demux  Outputs=2
  K_i : Gain  Gain=K_i  Multiplication=Matrix(K*u)
  K_i_13 : Gain  Gain=3.67146379600028
  K_i_31-22 : Gain  Gain=-1.50330201504916
  K_i_44 : Gain  Gain=6.55197651405933
  Manual Switch : ManualSwitch  CurrentSetting=0
  Mux : Mux
  Mux1 : Mux  Inputs=2
  Revert sign : Gain  Gain=-1
  u : Outport
  wires:
  K_i_13/1 -> Mux/1
  Manual Switch/1 -> u/1
  Demux/1 -> Mux1/1  "x"
  Demux/2 -> Mux1/2  "y"
  Demux/3 -> K_i_13/1  "z"
  Demux/4 -> K_i_44/1  "psi"
  Mux/1 -> Manual Switch/2
  K_i/1 -> Manual Switch/1
  K_i_44/1 -> Mux/4
  Revert sign/1 -> Mux/2
  int(e)/1 -> K_i/1, Demux/1
  Mux1/1 -> K_i_31-22/1
  K_i_31-22/1 -> Demux1/1
  Demux1/1 -> Mux/3
  Demux1/2 -> Revert sign/1

== system Masse_MultirotorSimHinf/K_p ==
  e : Inport
  Demux : Demux
  Demux1 : Demux  Outputs=2
  K_p : Gain  Gain=K_p  Multiplication=Matrix(K*u)
  K_p_13 : Gain  Gain=1.52717472910293
  K_p_31-22 : Gain  Gain=-0.500949072013311
  K_p_44 : Gain  Gain=1.18954454305298
  Manual Switch : ManualSwitch  CurrentSetting=0
  Mux : Mux
  Mux1 : Mux  Inputs=2
  Revert sign : Gain  Gain=-1
  u : Outport
  wires:
  e/1 -> Demux/1, K_p/1
  K_p/1 -> Manual Switch/1
  Mux/1 -> Manual Switch/2
  Manual Switch/1 -> u/1
  Revert sign/1 -> Mux/2
  Demux/2 -> Mux1/2  "y"
  Demux/1 -> Mux1/1  "x"
  Mux1/1 -> K_p_31-22/1
  K_p_13/1 -> Mux/1
  K_p_44/1 -> Mux/4
  Demux1/2 -> Revert sign/1
  Demux1/1 -> Mux/3
  Demux/4 -> K_p_44/1  "psi"
  K_p_31-22/1 -> Demux1/1
  Demux/3 -> K_p_13/1  "z"

== system Masse_MultirotorSimHinf/Logging buffer ==
  pwmIn : Inport
  pwmOut : Outport
  wires:
  pwmIn/1 -> pwmOut/1

== system Masse_MultirotorSimHinf/NWU to NED Position1 ==
  posNWU : Inport
  Multiply : Product  Inputs=**
  Position gain : Constant  Value=[1; -1; -1]
  posNED : Outport
  wires:
  posNWU/1 -> Multiply/1
  Multiply/1 -> posNED/1
  Position gain/1 -> Multiply/2

== system Masse_MultirotorSimHinf/NWU to NED Quaternion3 ==
  qNWU : Inport
  Multiply : Product  Inputs=**
  Quaternion gain : Constant  Value=[1; 1; -1; -1]
  qNED : Outport
  wires:
  Quaternion gain/1 -> Multiply/2
  Multiply/1 -> qNED/1
  qNWU/1 -> Multiply/1

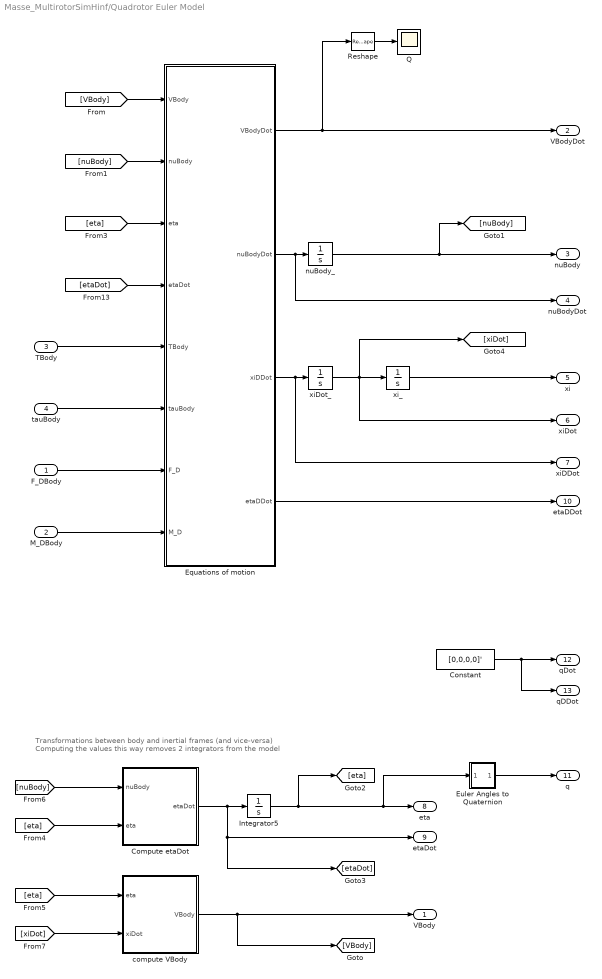
== system Masse_MultirotorSimHinf/Quadrotor Euler Model ==
  note: Transformations between body and inertial frames (and vice-versa)
      | Computing the values this way removes 2 integrators from the model
  F_DBody : Inport  Unit=N
  M_DBody : Inport  Port=2  Unit=N*m
  TBody : Inport  Port=3  Unit=N
  tauBody : Inport  Port=4  Unit=N*m
  Compute etaDot : MATLAB Function  TreatAsAtomicUnit=on
  Constant : Constant  Value=[0,0,0,0]'
  Equations of motion : MATLAB Function  TreatAsAtomicUnit=on
  Euler Angles to Quaternion : Subsystem  AncestorBlock=QuaternionLibrary/Euler Angles to Quaternion
      mask help: Convert vector of Euler angles to an orientation quaternion
      mask Help:
      | Convert vector of Euler angles
      | [roll, pitch, yaw]
      | to an orientation quaternion
      | [q1 q2 q3 q4]
      | where:
      | - q1 is the rotation in radians
      | - [q2 q3 q4] is the vector around which the rotation is performed)
      | 
      | Based on code from the PX4 firmware: https://github.com/PX4/Firmware
      mask Display: disp('E2Q')
  Integrator5 : Integrator  InitialCondition=Initial.ETA  ContinuousStateAttributes='eta'
  Q : Scope
  Reshape : Reshape  OutputDimensionality=Column vector (2-D)
  compute VBody : MATLAB Function  TreatAsAtomicUnit=on
  nuBody_ : Integrator  InitialCondition=Initial.NU_BODY  ContinuousStateAttributes='nuBody'
  xiDot_ : Integrator  InitialCondition=Initial.XI_DOT  ContinuousStateAttributes='xiDot'
  xi_ : Integrator  InitialCondition=Initial.XI  ContinuousStateAttributes='xi'
  VBody : Outport  Unit=m/s
  VBodyDot : Outport  Port=2  Unit=m/s^2
  nuBody : Outport  Port=3  Unit=rad/s
  nuBodyDot : Outport  Port=4  Unit=rad/s^2
  xi : Outport  Port=5  Unit=m
  xiDot : Outport  Port=6  Unit=m/s
  xiDDot : Outport  Port=7  Unit=m/s^2
  eta : Outport  Port=8  Unit=rad
  etaDot : Outport  Port=9  Unit=rad/s
  etaDDot : Outport  Port=10  Unit=rad/s^2
  q : Outport  Port=11
  qDot : Outport  Port=12
  qDDot : Outport  Port=13
  wires:
  Equations of motion/1(VBodyDot) -> Reshape/1, VBodyDot/1
  xi_/1 -> xi/1
  [nuBody] -> Equations of motion/2(nuBody)
  [VBody] -> Equations of motion/1(VBody)
  tauBody/1 -> Equations of motion/6(tauBody)
  TBody/1 -> Equations of motion/5(TBody)
  Equations of motion/3(xiDDot) -> xiDot_/1, xiDDot/1
  F_DBody/1 -> Equations of motion/7(F_D)
  M_DBody/1 -> Equations of motion/8(M_D)
  nuBody_/1 -> [nuBody], nuBody/1
  Equations of motion/2(nuBodyDot) -> nuBody_/1, nuBodyDot/1
  [eta] -> Equations of motion/3(eta)
  Equations of motion/4(etaDDot) -> etaDDot/1
  Reshape/1 -> Q/1
  xiDot_/1 -> xi_/1, [xiDot], xiDot/1
  [etaDot] -> Equations of motion/4(etaDot)
  [xiDot] -> compute VBody/2(xiDot)
  [nuBody] -> Compute etaDot/1(nuBody)
  [eta] -> compute VBody/1(eta)
  compute VBody/1(VBody) -> VBody/1, [VBody]
  [eta] -> Compute etaDot/2(eta)
  Compute etaDot/1(etaDot) -> etaDot/1, [etaDot], Integrator5/1
  Integrator5/1 -> Euler Angles to Quaternion/1(euler), eta/1, [eta]
  Euler Angles to Quaternion/1(quaternion) -> q/1
  Constant/1 -> qDDot/1, qDot/1
